simulink model "AMCLIB_BemfObsrvDQ_BAM_F16"  (Simulink 8.3)
settings: Solver=ode45  StartTime=0.0  StopTime=10.0  RelTol=1e-3
undefined symbols (not defined in the file): f16CC1sc_D, f16CC1sc_Q, f16CC2sc_D, f16CC2sc_Q, f16EGain, f16IGain, f16LowerLimit_D, f16LowerLimit_Q, f16UGain, f16UpperLimit_D, f16UpperLimit_Q, f16WIGain, s16Shift, u16NShift
settings Model: Creator=B37097  LastModifiedBy=B37097
settings DataIOCC: SignalLoggingSaveFormat=Dataset
settings DebuggingCC: UnderspecifiedInitializationDetection=Simplified  StateNameClashWarn=none
settings GRTTargetCC: CombineOutputUpdateFcns=on  GRTInterface=off

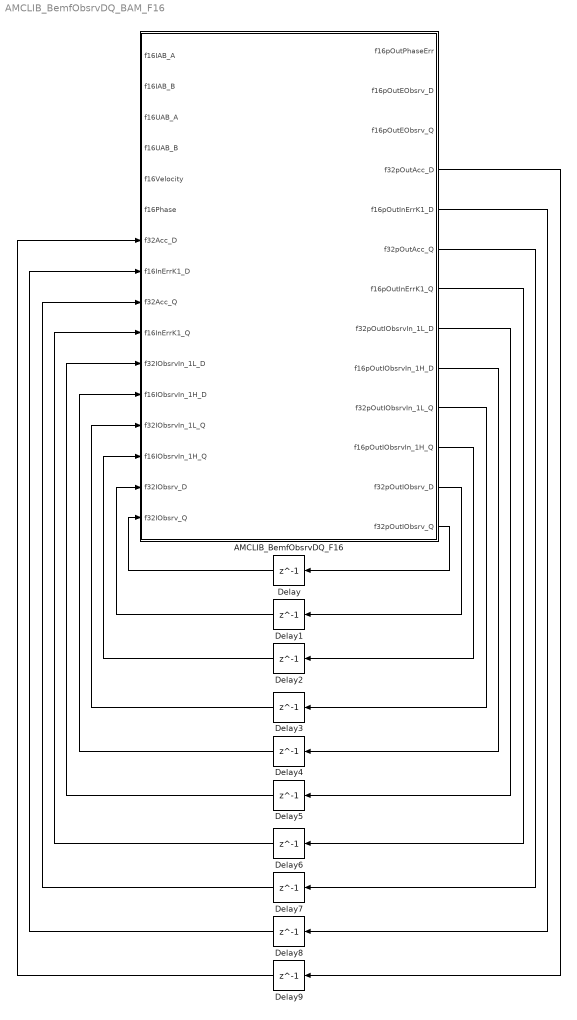
== system AMCLIB_BemfObsrvDQ_BAM_F16 ==
  AMCLIB_BemfObsrvDQ_F16 : Subsystem  mask(AMCLIB_BemfObsrvDQ_F16){f16IGain=f16IGain, f16UGain=f16UGain, f16WIGain=f16WIGain, f16EGain=f16EGain, s16Shift=s16Shift, f16CC1sc_D=f16CC1sc_D, f16CC1sc_Q=f16CC1sc_Q, f16CC2sc_D=f16CC2sc_D, f16CC2sc_Q=f16CC2sc_Q, f16UpperLimit_D=f16UpperLimit_D, f16UpperLimit_Q=f16UpperLimit_Q, f16LowerLimit_D=f16LowerLimit_D, f16LowerLimit_Q=f16LowerLimit_Q, u16NShift=u16NShift}
      mask help: Bit accurate model of back-EMF observer DQ in 16-bit fixed-point implementation.
      mask init:
      | pos = get_param(gcb, 'Position');width = pos(3) - pos(1); height = pos(4) - pos(2);tX=width/2;tY=height*0.9;
      mask Display: color('black');port_label('input',1,'f16IAB_A');port_label('input',2,'f16IAB_B');port_label('input',3,'f16UAB_A');port_label('input',4,'f16UAB_B');port_label('input',5,'f16Velocity');port_label('input',6,'f16Phase');port_label('input',7,'f32Acc_D');port_label('input',8,'f16InErrK1_D');port_label('input',9,'f32Acc_Q');port_label('input',10,'f16InErrK1_Q');port_label('input',11,'f32IObsrvIn_1L_D');port_label('input',12,'f16IObsrvIn_1H_D');port_label('input',13,'f32IObsrvIn_1L_Q');port_label('input',14,'f16IObsrvIn_1H_Q');port_label('input',15,'f32IObsrv_D');port_label('input',16,'f32IObsrv_Q');port_label('output',1,'f16pOutPhaseErr');port_label('output',2,'f16pOutEObsrv_D');port_label('output',3,'f16pOutEObsrv_Q');port_label('output',4,'f32pOutAcc_D');port_label('output',5,'f16pOutInErrK1_D');port_label('output',6,'f32pOutAcc_Q');port_label('output',7,'f16pOutInErrK1_Q');port_label('output',8,'f32pOutIObsrvIn_1L_D');port_label('output',9,'f16pOutIObsrvIn_1H_D');port_label('output',10,'f32pOutIObsrvIn_1L_Q');port_label('output',11,'f16pOutIObsrvIn_1H_Q');port_label('output',12,'f32pOutIObsrv_D');port_label('output',13,'f32pOutIObsrv_Q');color('black');disp('AMCLIB_BemfObsrvDQ_F16');color('blue');text(tX,tY, 'BAM', 'horizontalAlignment', 'center');
  Delay{,1..9} (10 alike) : Delay  DelayLength=1  InitialCondition=0
  wires:
  AMCLIB_BemfObsrvDQ_F16/13(f32pOutIObsrv_Q) -> Delay/1
  Delay/1 -> AMCLIB_BemfObsrvDQ_F16/16(f32IObsrv_Q)
  AMCLIB_BemfObsrvDQ_F16/12(f32pOutIObsrv_D) -> Delay1/1
  Delay1/1 -> AMCLIB_BemfObsrvDQ_F16/15(f32IObsrv_D)
  AMCLIB_BemfObsrvDQ_F16/11(f16pOutIObsrvIn_1H_Q) -> Delay2/1
  Delay2/1 -> AMCLIB_BemfObsrvDQ_F16/14(f16IObsrvIn_1H_Q)
  AMCLIB_BemfObsrvDQ_F16/10(f32pOutIObsrvIn_1L_Q) -> Delay3/1
  Delay3/1 -> AMCLIB_BemfObsrvDQ_F16/13(f32IObsrvIn_1L_Q)
  AMCLIB_BemfObsrvDQ_F16/9(f16pOutIObsrvIn_1H_D) -> Delay4/1
  Delay4/1 -> AMCLIB_BemfObsrvDQ_F16/12(f16IObsrvIn_1H_D)
  AMCLIB_BemfObsrvDQ_F16/8(f32pOutIObsrvIn_1L_D) -> Delay5/1
  Delay5/1 -> AMCLIB_BemfObsrvDQ_F16/11(f32IObsrvIn_1L_D)
  AMCLIB_BemfObsrvDQ_F16/7(f16pOutInErrK1_Q) -> Delay6/1
  Delay6/1 -> AMCLIB_BemfObsrvDQ_F16/10(f16InErrK1_Q)
  AMCLIB_BemfObsrvDQ_F16/6(f32pOutAcc_Q) -> Delay7/1
  Delay7/1 -> AMCLIB_BemfObsrvDQ_F16/9(f32Acc_Q)
  AMCLIB_BemfObsrvDQ_F16/5(f16pOutInErrK1_D) -> Delay8/1
  Delay8/1 -> AMCLIB_BemfObsrvDQ_F16/8(f16InErrK1_D)
  AMCLIB_BemfObsrvDQ_F16/4(f32pOutAcc_D) -> Delay9/1
  Delay9/1 -> AMCLIB_BemfObsrvDQ_F16/7(f32Acc_D)

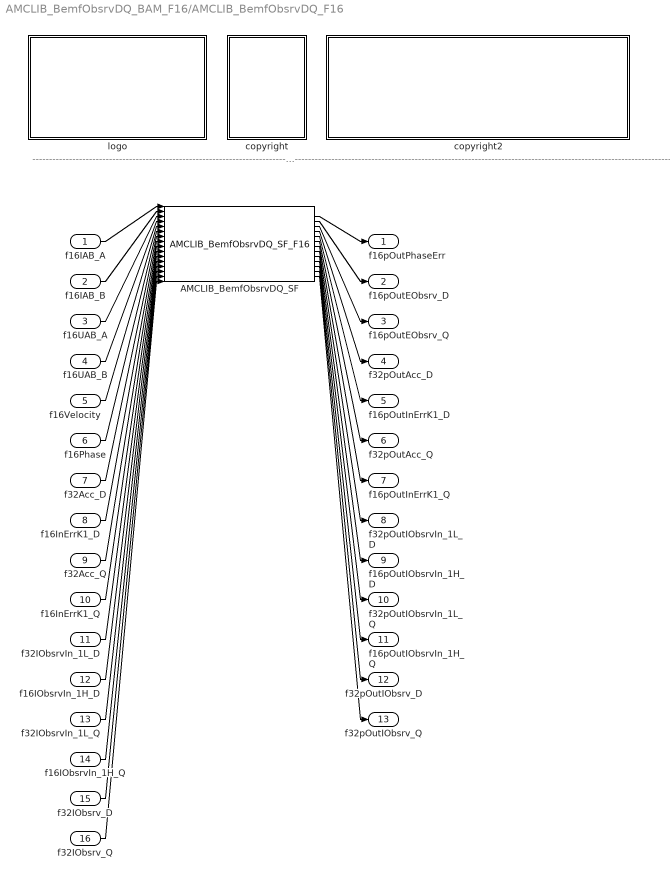
== system AMCLIB_BemfObsrvDQ_BAM_F16/AMCLIB_BemfObsrvDQ_F16 ==
  note: ---------------------------------------------------------------------------------------------------------------------------------------------------------------------------------------------------
  f16IAB_A : Inport
  f16IAB_B : Inport  Port=2
  f16UAB_A : Inport  Port=3
  f16UAB_B : Inport  Port=4
  f16Velocity : Inport  Port=5
  f16Phase : Inport  Port=6
  f32Acc_D : Inport  Port=7
  f16InErrK1_D : Inport  Port=8
  f32Acc_Q : Inport  Port=9
  f16InErrK1_Q : Inport  Port=10
  f32IObsrvIn_1L_D : Inport  Port=11
  f16IObsrvIn_1H_D : Inport  Port=12
  f32IObsrvIn_1L_Q : Inport  Port=13
  f16IObsrvIn_1H_Q : Inport  Port=14
  f32IObsrv_D : Inport  Port=15
  f32IObsrv_Q : Inport  Port=16
  AMCLIB_BemfObsrvDQ_SF : S-Function  FunctionName=AMCLIB_BemfObsrvDQ_SF_F16  Parameters=f16IGain,f16UGain,f16WIGain,f16EGain,s16Shift,f16CC1sc_D,f16CC1sc_Q,f16CC2sc_D,f16CC2sc_Q,f16UpperLimit_D,f16UpperLimit_Q,f16LowerLimit_D,f16LowerLimit_Q,u16NShift  EnableBusSupport=off
  copyright : Subsystem
      mask Display: text(10,90,'FILE:');text(10,75,'DESRIPTION:');text(10,60,'COPYRIGHT:');text(10,45,'VERSION:');text(10,30,'DATE:')
  copyright2 : Subsystem
      mask Display: text(10,90,'AMCLIB_BemfObsrvDQ_BAM_F16.mdl');text(10,75,'PMSM back-EMF observer DQ.');text(10,60,'NXP');text(10,45,'1.0');text(10,30,'26-Oct-2016');
  logo : Subsystem
      mask Display: image(imread('logo.jpg'))
  f16pOutPhaseErr : Outport
  f16pOutEObsrv_D : Outport  Port=2
  f16pOutEObsrv_Q : Outport  Port=3
  f32pOutAcc_D : Outport  Port=4
  f16pOutInErrK1_D : Outport  Port=5
  f32pOutAcc_Q : Outport  Port=6
  f16pOutInErrK1_Q : Outport  Port=7
  f32pOutIObsrvIn_1L_D : Outport  Port=8
  f16pOutIObsrvIn_1H_D : Outport  Port=9
  f32pOutIObsrvIn_1L_Q : Outport  Port=10
  f16pOutIObsrvIn_1H_Q : Outport  Port=11
  f32pOutIObsrv_D : Outport  Port=12
  f32pOutIObsrv_Q : Outport  Port=13
  wires:
  f16IAB_A/1 -> AMCLIB_BemfObsrvDQ_SF/1
  f16IAB_B/1 -> AMCLIB_BemfObsrvDQ_SF/2
  f16UAB_A/1 -> AMCLIB_BemfObsrvDQ_SF/3
  f16UAB_B/1 -> AMCLIB_BemfObsrvDQ_SF/4
  f16Velocity/1 -> AMCLIB_BemfObsrvDQ_SF/5
  f16Phase/1 -> AMCLIB_BemfObsrvDQ_SF/6
  f32Acc_D/1 -> AMCLIB_BemfObsrvDQ_SF/7
  f16InErrK1_D/1 -> AMCLIB_BemfObsrvDQ_SF/8
  f32Acc_Q/1 -> AMCLIB_BemfObsrvDQ_SF/9
  f16InErrK1_Q/1 -> AMCLIB_BemfObsrvDQ_SF/10
  f32IObsrvIn_1L_D/1 -> AMCLIB_BemfObsrvDQ_SF/11
  f16IObsrvIn_1H_D/1 -> AMCLIB_BemfObsrvDQ_SF/12
  f32IObsrvIn_1L_Q/1 -> AMCLIB_BemfObsrvDQ_SF/13
  f16IObsrvIn_1H_Q/1 -> AMCLIB_BemfObsrvDQ_SF/14
  f32IObsrv_D/1 -> AMCLIB_BemfObsrvDQ_SF/15
  f32IObsrv_Q/1 -> AMCLIB_BemfObsrvDQ_SF/16
  AMCLIB_BemfObsrvDQ_SF/1 -> f16pOutPhaseErr/1
  AMCLIB_BemfObsrvDQ_SF/2 -> f16pOutEObsrv_D/1
  AMCLIB_BemfObsrvDQ_SF/3 -> f16pOutEObsrv_Q/1
  AMCLIB_BemfObsrvDQ_SF/4 -> f32pOutAcc_D/1
  AMCLIB_BemfObsrvDQ_SF/5 -> f16pOutInErrK1_D/1
  AMCLIB_BemfObsrvDQ_SF/6 -> f32pOutAcc_Q/1
  AMCLIB_BemfObsrvDQ_SF/7 -> f16pOutInErrK1_Q/1
  AMCLIB_BemfObsrvDQ_SF/8 -> f32pOutIObsrvIn_1L_D/1
  AMCLIB_BemfObsrvDQ_SF/9 -> f16pOutIObsrvIn_1H_D/1
  AMCLIB_BemfObsrvDQ_SF/10 -> f32pOutIObsrvIn_1L_Q/1
  AMCLIB_BemfObsrvDQ_SF/11 -> f16pOutIObsrvIn_1H_Q/1
  AMCLIB_BemfObsrvDQ_SF/12 -> f32pOutIObsrv_D/1
  AMCLIB_BemfObsrvDQ_SF/13 -> f32pOutIObsrv_Q/1

== system AMCLIB_BemfObsrvDQ_BAM_F16/AMCLIB_BemfObsrvDQ_F16/copyright ==

== system AMCLIB_BemfObsrvDQ_BAM_F16/AMCLIB_BemfObsrvDQ_F16/copyright2 ==

== system AMCLIB_BemfObsrvDQ_BAM_F16/AMCLIB_BemfObsrvDQ_F16/logo ==
